simulink model "mpulse_vector_SimOnly_1"  (Simulink 6.3)
settings: Solver=ode45  StartTime=0.0  StopTime=0  RelTol=1e-3
settings Model: Creator=zren  LastModifiedBy=mshakeri  ExtModeEnableOpenProtocolUploading=on  ExtModeOpenProtocolUploadingEqualLengthVectors=off  ExtModeAutoUpdateStatusClock=off  StrictBusMsg=ErrorLevel1
settings OptimizationCC: BlockReduction=off  BooleanDataType=off  InlineParams=on
settings DebuggingCC: AlgebraicLoopMsg=error  SignalResolutionControl=UseLocalSettings  SolverPrmCheckMsg=none  UnknownTsInhSupMsg=none  ModelReferenceDataLoggingMessage=none
settings HardwareCC: TargetUnknown=on
settings ModelReferenceCC: UpdateModelReferenceTargets=IfOutOfDate
settings RTWCC: GenerateReport=on  LaunchReport=on

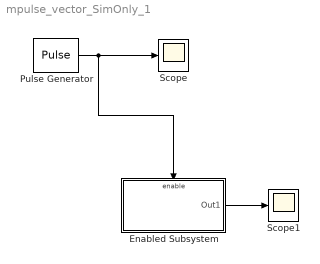
== system mpulse_vector_SimOnly_1 ==
  Enabled Subsystem : Subsystem  TreatAsAtomicUnit=on
  Pulse Generator : DiscretePulseGenerator  PulseType=Time based  Amplitude=[1, 2, 3]  PulseWidth=50  PhaseDelay=[ 0.2,0.5,0.7]
  Scope : Scope
      settings: SaveName=scopeout1
  Scope1 : Scope
      settings: SaveName=scopeout2
  wires:
  Pulse Generator/1 -> Scope/1, Enabled Subsystem/Enable
  Enabled Subsystem/1(Out1) -> Scope1/1

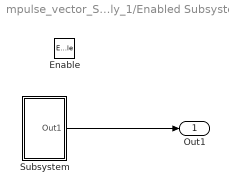
== system mpulse_vector_SimOnly_1/Enabled Subsystem ==
  Enable : EnablePort
  Subsystem : Subsystem  TreatAsAtomicUnit=on
  Out1 : Outport
  wires:
  Subsystem/1(Out1) -> Out1/1

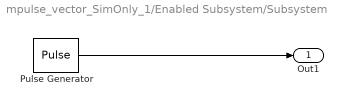
== system mpulse_vector_SimOnly_1/Enabled Subsystem/Subsystem ==
  Pulse Generator : DiscretePulseGenerator  PulseType=Time based  Amplitude=[6, 15]  Period=0.3  PulseWidth=50  PhaseDelay=-0.15
  Out1 : Outport
  wires:
  Pulse Generator/1 -> Out1/1
